simulink model "SecRwLtStBkReclnIsPosChk"  (R2024b)
settings: Solver=FixedStepDiscrete  StartTime=0.0  StopTime=10.0  FixedStep=0.01  RelTol=1e-3
undefined symbols (not defined in the file or in its folder): KeSMSuSecRwStBackPosDelta_Val, KeSMSuSecRwStBackPosTolr_Val, KeSMSuVehicleModelConfig_Val
libraries: StIsPosChkLib x13, simulink x7
(part 1 of 2)
settings Model: Creator=sn2xws  LastModifiedBy=sn55gm
settings Model: ModifiedHistory=|
  | 2023.8.1 V2.0.0 CR421790 增加模式21-26
  | 2024.3.14
  | V2.3.0
  | Bug 813950 童锁Lock，Mode1_Easy Entry Mode 不应调用失败
  | 2024.5.7 557 eze模式变更
  | 2024.7.8 V3.0.1 557模式流程V1.9
  | 2024.8.20 V3.0.2 Md32isposZone不看二排靠背
  | 2024.9.4 V3.0.3 增加Md56大四座模式（替代MD25）注释掉不用的模式
  | 2024.9.18 V3.0.4 Md27误注释恢复
  | 2024.12.17 V3.0.5 Md57 Md58 报失败问题修复
  | 2025.5.20 V3.12.0 童锁 Md56应报成功
  | 25.7.1 V3.13.0 新增Md61 Md62
settings SolverCC: AlgebraicLoopSolver=TrustRegion
settings DataIOCC: SaveFormat=StructureWithTime  ReturnWorkspaceOutputs=off
settings OptimizationCC: DefaultParameterBehavior=Inlined  EnhancedBackFolding=on  PassReuseOutputArgsAs=Individual arguments  ZeroExternalMemoryAtStartup=off  ZeroInternalMemoryAtStartup=off  OptimizeBlockOrder=speed  DifferentSizesBufferReuse=on  OptimizationCustomize=off  EfficientTunableParamExpr=on
settings DebuggingCC: ParameterTunabilityLossMsg=error  UnconnectedInputMsg=warning  UnconnectedOutputMsg=warning  UnconnectedLineMsg=warning  ArithmeticOperatorsInVariantConditions=warning
settings ModelReferenceCC: EnableRefExpFcnMdlSchedulingChecks=on  ModelReferenceNumInstancesAllowed=Single
settings SFSimCC: MATLABDynamicMemAlloc=off  CustomCodeUndefinedFunction=UseInterfaceOnly
settings RTWCC: Description=AUTOSAR  SystemTargetFile=autosar.tlc  GenCodeOnly=on  TemplateMakefile=ert_default_tmf  GenerateReport=on  IncludeHyperlinkInReport=on  LaunchReport=on  DataTypeReplacement=CDataTypesFixedWidth  GenerateTraceInfo=on  GenerateTraceReport=on  GenerateTraceReportSl=on  GenerateTraceReportSf=on  GenerateTraceReportEml=on  GenerateCodeMetricsReport=on  GPUComputeCapability=3.5
settings CodeAppCC: ForceParamTrailComments=on  IgnoreCustomStorageClasses=off  OperatorAnnotations=on  SimulinkDataObjDesc=on  SFDataObjDesc=on  InsertBlockDesc=on
settings STFCustomTargetCC: TargetLangStandard=C99 (ISO)  MultiwordLength=256  ParMdlRefBuildCompliant=on  CompOptLevelCompliant=on  IncludeMdlTerminateFcn=off  CombineOutputUpdateFcns=on  SuppressErrorStatus=on  ERTCustomFileBanners=on  SupportNonFinite=off  SupportComplex=off  SupportContinuousTime=off  SupportNonInlinedSFcns=off  RemoveResetFunc=on  MATLABClassNameForMDSCustomization=Simulink.SoftwareTarget.ERTCustomization  AutosarCompliant=on  UseToolchainInfoCompliant=on  LookupTableObjectStructAxisOrder=2,1,3,4,...  LUTObjectStructOrderEvenSpacing=Size,Table,Breakpoints  SystemTargetFile=autosar.tlc
settings ERTTargetCC: TargetLangStandard=C99 (ISO)  ConcurrentExecutionCompliant=off  IncludeMdlTerminateFcn=off  SuppressErrorStatus=on  SupportNonFinite=off  SupportComplex=off  ModelStepFunctionPrototypeControlCompliant=off  CPPClassGenCompliant=off  AutosarCompliant=on  LookupTableObjectStructAxisOrder=2,1,3,4,...  LUTObjectStructOrderEvenSpacing=Size,Table,Breakpoints  ERTCustomFileTemplate=example_file_process.tlc  ERTFilePackagingFormat=Compact  BooleanTrueId=TRUE  BooleanFalseId=FALSE  DynamicArrayContainerType=coder::array

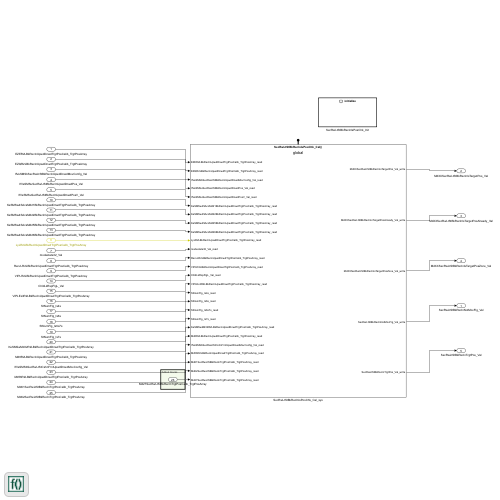
[thumbnail: Simulink's stored preview of the top-level diagram]
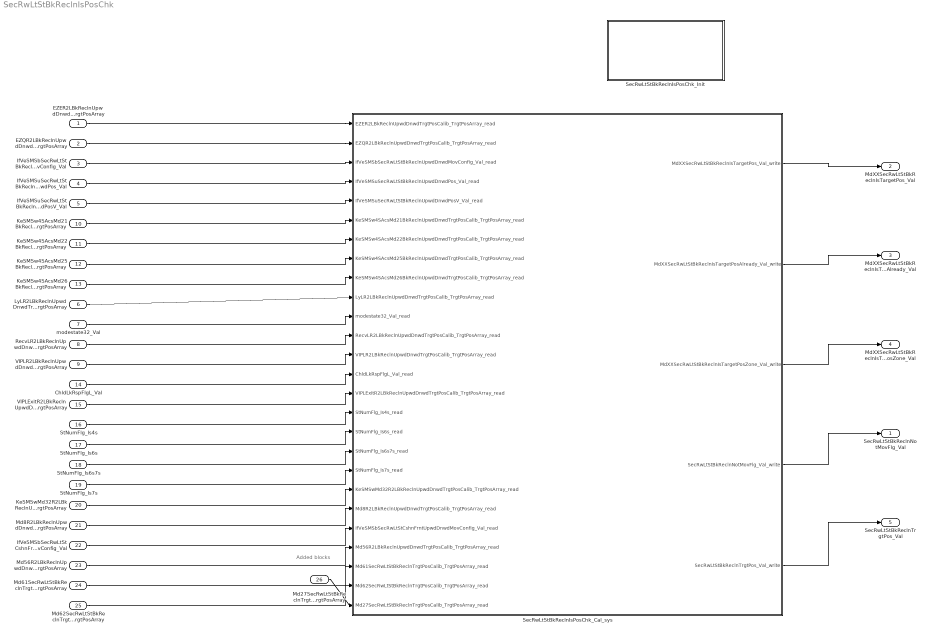
== system SecRwLtStBkReclnIsPosChk ==
  note: Added blocks
  EZER2LBkReclnUpwdDnwdTrgtPosCalib_TrgtPosArray : Inport  Description=|  OutDataTypeStr=uint16  PortDimensions=3
      | 0:Pos
      | 1:Max
      | 2:Min
  EZQR2LBkReclnUpwdDnwdTrgtPosCalib_TrgtPosArray : Inport  Description=|  Port=2  OutDataTypeStr=uint16  PortDimensions=3
      | 0:Pos
      | 1:Max
      | 2:Min
  IfVeSMSbSecRwLtStBkReclnUpwdDnwdMovConfig_Val : Inport  Port=3  OutDataTypeStr=boolean  PortDimensions=1
  IfVeSMSuSecRwLtStBkReclnUpwdDnwdPos_Val : Inport  Port=4  OutDataTypeStr=uint16  PortDimensions=1
  IfVeSMSuSecRwLtStBkReclnUpwdDnwdPosV_Val : Inport  Port=5  OutDataTypeStr=boolean  PortDimensions=1
  LyLR2LBkReclnUpwdDnwdTrgtPosCalib_TrgtPosArray : Inport  Description=|  Port=6  OutDataTypeStr=uint16  PortDimensions=3
      | 0:Pos
      | 1:Max
      | 2:Min
  modestate32_Val : Inport  Port=7  OutDataTypeStr=uint32  PortDimensions=1
  RecvLR2LBkReclnUpwdDnwdTrgtPosCalib_TrgtPosArray : Inport  Description=|  Port=8  OutDataTypeStr=uint16  PortDimensions=3
      | 0:Pos
      | 1:Max
      | 2:Min
  VIPLR2LBkReclnUpwdDnwdTrgtPosCalib_TrgtPosArray : Inport  Description=|  Port=9  OutDataTypeStr=uint16  PortDimensions=3
      | 0:Pos
      | 1:Max
      | 2:Min
  KeSMSw4SAcsMd21BkReclnUpwdDnwdTrgtPosCalib_TrgtPosArray : Inport  Description=|  Port=10  OutDataTypeStr=uint16  PortDimensions=3
      | 0:Pos
      | 1:Max
      | 2:Min
  KeSMSw4SAcsMd22BkReclnUpwdDnwdTrgtPosCalib_TrgtPosArray : Inport  Description=|  Port=11  OutDataTypeStr=uint16  PortDimensions=3
      | 0:Pos
      | 1:Max
      | 2:Min
  KeSMSw4SAcsMd25BkReclnUpwdDnwdTrgtPosCalib_TrgtPosArray : Inport  Description=|  Port=12  OutDataTypeStr=uint16  PortDimensions=3
      | 0:Pos
      | 1:Max
      | 2:Min
  KeSMSw4SAcsMd26BkReclnUpwdDnwdTrgtPosCalib_TrgtPosArray : Inport  Description=|  Port=13  OutDataTypeStr=uint16  PortDimensions=3
      | 0:Pos
      | 1:Max
      | 2:Min
  ChldLkRspFlgL_Val : Inport  Port=14  OutDataTypeStr=boolean  PortDimensions=1
  VIPLExitR2LBkReclnUpwdDnwdTrgtPosCalib_TrgtPosArray : Inport  Description=|  Port=15  OutDataTypeStr=uint16  PortDimensions=3
      | 0:Pos
      | 1:Max
      | 2:Min
  StNumFlg_Is4s : Inport  Port=16  OutDataTypeStr=boolean  PortDimensions=1
  StNumFlg_Is6s : Inport  Port=17  OutDataTypeStr=boolean  PortDimensions=1
  StNumFlg_Is6s7s : Inport  Port=18  OutDataTypeStr=boolean  PortDimensions=1
  StNumFlg_Is7s : Inport  Port=19  OutDataTypeStr=boolean  PortDimensions=1
  KeSMSwMd32R2LBkReclnUpwdDnwdTrgtPosCalib_TrgtPosArray : Inport  Description=|  Port=20  OutDataTypeStr=uint16  PortDimensions=3
      | 0:Pos
      | 1:Max
      | 2:Min
  Md8R2LBkReclnUpwdDnwdTrgtPosCalib_TrgtPosArray : Inport  Description=|  Port=21  OutDataTypeStr=uint16  PortDimensions=3
      | 0:Pos
      | 1:Max
      | 2:Min
  IfVeSMSbSecRwLtStCshnFrntUpwdDnwdMovConfig_Val : Inport  Port=22  OutDataTypeStr=boolean  PortDimensions=1
  Md56R2LBkReclnUpwdDnwdTrgtPosCalib_TrgtPosArray : Inport  Description=|  Port=23  OutDataTypeStr=uint16  PortDimensions=3
      | 0:Pos
      | 1:Max
      | 2:Min
  Md61SecRwLtStBkReclnTrgtPosCalib_TrgtPosArray : Inport  Description=|  Port=24  OutDataTypeStr=uint16  PortDimensions=3
      | 0:Pos
      | 1:Max
      | 2:Min
  Md62SecRwLtStBkReclnTrgtPosCalib_TrgtPosArray : Inport  Description=|  Port=25  OutDataTypeStr=uint16  PortDimensions=3
      | 0:Pos
      | 1:Max
      | 2:Min
  Md27SecRwLtStBkReclnTrgtPosCalib_TrgtPosArray : Inport  Description=|  Port=26  OutDataTypeStr=uint16  PortDimensions=3
      | 0:Pos
      | 1:Max
      | 2:Min
  SecRwLtStBkReclnIsPosChk_Cal_sys : Subsystem
  SecRwLtStBkReclnIsPosChk_Init : Subsystem
  SecRwLtStBkReclnNotMovFlg_Val : Outport  OutDataTypeStr=boolean  PortDimensions=1  VectorParamsAs1DForOutWhenUnconnected=off
  MdXXSecRwLtStBkReclnIsTargetPos_Val : Outport  Port=2  OutDataTypeStr=uint32  PortDimensions=1  VectorParamsAs1DForOutWhenUnconnected=off
  MdXXSecRwLtStBkReclnIsTargetPosAlready_Val : Outport  Port=3  OutDataTypeStr=uint32  PortDimensions=1  VectorParamsAs1DForOutWhenUnconnected=off
  MdXXSecRwLtStBkReclnIsTargetPosZone_Val : Outport  Port=4  OutDataTypeStr=uint32  PortDimensions=1  VectorParamsAs1DForOutWhenUnconnected=off
  SecRwLtStBkReclnTrgtPos_Val : Outport  Port=5  OutDataTypeStr=uint16  PortDimensions=1  VectorParamsAs1DForOutWhenUnconnected=off
  wires:
  EZER2LBkReclnUpwdDnwdTrgtPosCalib_TrgtPosArray/1 -> SecRwLtStBkReclnIsPosChk_Cal_sys/1(EZER2LBkReclnUpwdDnwdTrgtPosCalib_TrgtPosArray_read)
  EZQR2LBkReclnUpwdDnwdTrgtPosCalib_TrgtPosArray/1 -> SecRwLtStBkReclnIsPosChk_Cal_sys/2(EZQR2LBkReclnUpwdDnwdTrgtPosCalib_TrgtPosArray_read)
  IfVeSMSbSecRwLtStBkReclnUpwdDnwdMovConfig_Val/1 -> SecRwLtStBkReclnIsPosChk_Cal_sys/3(IfVeSMSbSecRwLtStBkReclnUpwdDnwdMovConfig_Val_read)
  IfVeSMSuSecRwLtStBkReclnUpwdDnwdPos_Val/1 -> SecRwLtStBkReclnIsPosChk_Cal_sys/4(IfVeSMSuSecRwLtStBkReclnUpwdDnwdPos_Val_read)
  IfVeSMSuSecRwLtStBkReclnUpwdDnwdPosV_Val/1 -> SecRwLtStBkReclnIsPosChk_Cal_sys/5(IfVeSMSuSecRwLtStBkReclnUpwdDnwdPosV_Val_read)
  LyLR2LBkReclnUpwdDnwdTrgtPosCalib_TrgtPosArray/1 -> SecRwLtStBkReclnIsPosChk_Cal_sys/10(LyLR2LBkReclnUpwdDnwdTrgtPosCalib_TrgtPosArray_read)
  modestate32_Val/1 -> SecRwLtStBkReclnIsPosChk_Cal_sys/11(modestate32_Val_read)
  RecvLR2LBkReclnUpwdDnwdTrgtPosCalib_TrgtPosArray/1 -> SecRwLtStBkReclnIsPosChk_Cal_sys/12(RecvLR2LBkReclnUpwdDnwdTrgtPosCalib_TrgtPosArray_read)
  VIPLR2LBkReclnUpwdDnwdTrgtPosCalib_TrgtPosArray/1 -> SecRwLtStBkReclnIsPosChk_Cal_sys/13(VIPLR2LBkReclnUpwdDnwdTrgtPosCalib_TrgtPosArray_read)
  SecRwLtStBkReclnIsPosChk_Cal_sys/1(MdXXSecRwLtStBkReclnIsTargetPos_Val_write) -> MdXXSecRwLtStBkReclnIsTargetPos_Val/1
  SecRwLtStBkReclnIsPosChk_Cal_sys/2(MdXXSecRwLtStBkReclnIsTargetPosAlready_Val_write) -> MdXXSecRwLtStBkReclnIsTargetPosAlready_Val/1
  SecRwLtStBkReclnIsPosChk_Cal_sys/3(MdXXSecRwLtStBkReclnIsTargetPosZone_Val_write) -> MdXXSecRwLtStBkReclnIsTargetPosZone_Val/1
  SecRwLtStBkReclnIsPosChk_Cal_sys/4(SecRwLtStBkReclnNotMovFlg_Val_write) -> SecRwLtStBkReclnNotMovFlg_Val/1
  SecRwLtStBkReclnIsPosChk_Cal_sys/5(SecRwLtStBkReclnTrgtPos_Val_write) -> SecRwLtStBkReclnTrgtPos_Val/1
  KeSMSw4SAcsMd21BkReclnUpwdDnwdTrgtPosCalib_TrgtPosArray/1 -> SecRwLtStBkReclnIsPosChk_Cal_sys/6(KeSMSw4SAcsMd21BkReclnUpwdDnwdTrgtPosCalib_TrgtPosArray_read)
  KeSMSw4SAcsMd22BkReclnUpwdDnwdTrgtPosCalib_TrgtPosArray/1 -> SecRwLtStBkReclnIsPosChk_Cal_sys/7(KeSMSw4SAcsMd22BkReclnUpwdDnwdTrgtPosCalib_TrgtPosArray_read)
  KeSMSw4SAcsMd25BkReclnUpwdDnwdTrgtPosCalib_TrgtPosArray/1 -> SecRwLtStBkReclnIsPosChk_Cal_sys/8(KeSMSw4SAcsMd25BkReclnUpwdDnwdTrgtPosCalib_TrgtPosArray_read)
  KeSMSw4SAcsMd26BkReclnUpwdDnwdTrgtPosCalib_TrgtPosArray/1 -> SecRwLtStBkReclnIsPosChk_Cal_sys/9(KeSMSw4SAcsMd26BkReclnUpwdDnwdTrgtPosCalib_TrgtPosArray_read)
  ChldLkRspFlgL_Val/1 -> SecRwLtStBkReclnIsPosChk_Cal_sys/14(ChldLkRspFlgL_Val_read)
  VIPLExitR2LBkReclnUpwdDnwdTrgtPosCalib_TrgtPosArray/1 -> SecRwLtStBkReclnIsPosChk_Cal_sys/15(VIPLExitR2LBkReclnUpwdDnwdTrgtPosCalib_TrgtPosArray_read)
  StNumFlg_Is4s/1 -> SecRwLtStBkReclnIsPosChk_Cal_sys/16(StNumFlg_Is4s_read)
  StNumFlg_Is6s/1 -> SecRwLtStBkReclnIsPosChk_Cal_sys/17(StNumFlg_Is6s_read)
  StNumFlg_Is6s7s/1 -> SecRwLtStBkReclnIsPosChk_Cal_sys/18(StNumFlg_Is6s7s_read)
  StNumFlg_Is7s/1 -> SecRwLtStBkReclnIsPosChk_Cal_sys/19(StNumFlg_Is7s_read)
  KeSMSwMd32R2LBkReclnUpwdDnwdTrgtPosCalib_TrgtPosArray/1 -> SecRwLtStBkReclnIsPosChk_Cal_sys/20(KeSMSwMd32R2LBkReclnUpwdDnwdTrgtPosCalib_TrgtPosArray_read)
  Md8R2LBkReclnUpwdDnwdTrgtPosCalib_TrgtPosArray/1 -> SecRwLtStBkReclnIsPosChk_Cal_sys/21(Md8R2LBkReclnUpwdDnwdTrgtPosCalib_TrgtPosArray_read)
  IfVeSMSbSecRwLtStCshnFrntUpwdDnwdMovConfig_Val/1 -> SecRwLtStBkReclnIsPosChk_Cal_sys/22(IfVeSMSbSecRwLtStCshnFrntUpwdDnwdMovConfig_Val_read)
  Md56R2LBkReclnUpwdDnwdTrgtPosCalib_TrgtPosArray/1 -> SecRwLtStBkReclnIsPosChk_Cal_sys/23(Md56R2LBkReclnUpwdDnwdTrgtPosCalib_TrgtPosArray_read)
  Md61SecRwLtStBkReclnTrgtPosCalib_TrgtPosArray/1 -> SecRwLtStBkReclnIsPosChk_Cal_sys/24(Md61SecRwLtStBkReclnTrgtPosCalib_TrgtPosArray_read)
  Md62SecRwLtStBkReclnTrgtPosCalib_TrgtPosArray/1 -> SecRwLtStBkReclnIsPosChk_Cal_sys/25(Md62SecRwLtStBkReclnTrgtPosCalib_TrgtPosArray_read)
  Md27SecRwLtStBkReclnTrgtPosCalib_TrgtPosArray/1 -> SecRwLtStBkReclnIsPosChk_Cal_sys/26(Md27SecRwLtStBkReclnTrgtPosCalib_TrgtPosArray_read)

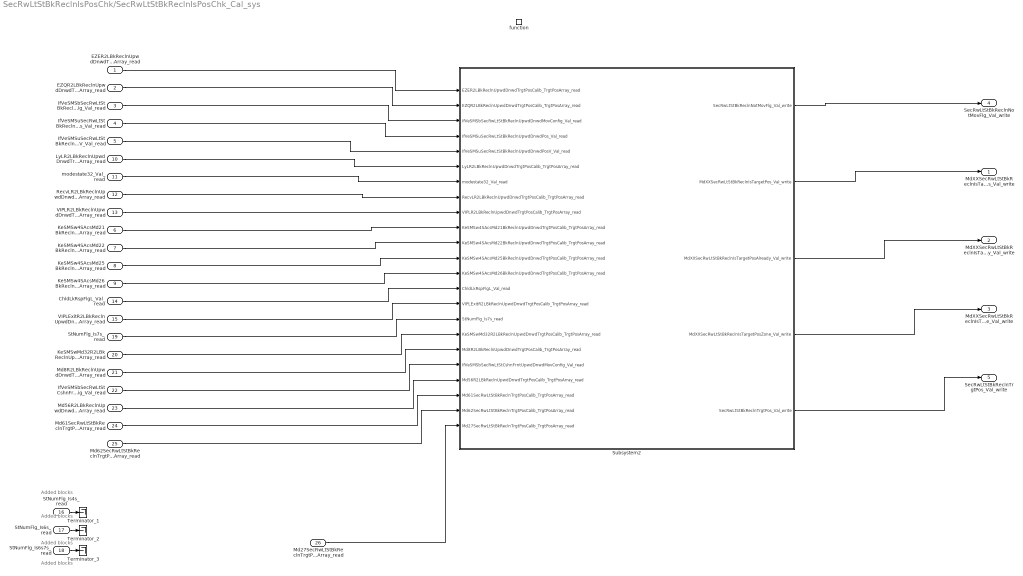
== system SecRwLtStBkReclnIsPosChk/SecRwLtStBkReclnIsPosChk_Cal_sys ==
  note: Added blocks
  note: Added blocks
  note: Added blocks
  note: Added blocks
  EZER2LBkReclnUpwdDnwdTrgtPosCalib_TrgtPosArray_read : Inport
  EZQR2LBkReclnUpwdDnwdTrgtPosCalib_TrgtPosArray_read : Inport  Port=2
  IfVeSMSbSecRwLtStBkReclnUpwdDnwdMovConfig_Val_read : Inport  Port=3
  IfVeSMSuSecRwLtStBkReclnUpwdDnwdPos_Val_read : Inport  Port=4
  IfVeSMSuSecRwLtStBkReclnUpwdDnwdPosV_Val_read : Inport  Port=5
  KeSMSw4SAcsMd21BkReclnUpwdDnwdTrgtPosCalib_TrgtPosArray_read : Inport  Port=6
  KeSMSw4SAcsMd22BkReclnUpwdDnwdTrgtPosCalib_TrgtPosArray_read : Inport  Port=7
  KeSMSw4SAcsMd25BkReclnUpwdDnwdTrgtPosCalib_TrgtPosArray_read : Inport  Port=8
  KeSMSw4SAcsMd26BkReclnUpwdDnwdTrgtPosCalib_TrgtPosArray_read : Inport  Port=9
  LyLR2LBkReclnUpwdDnwdTrgtPosCalib_TrgtPosArray_read : Inport  Port=10
  modestate32_Val_read : Inport  Port=11
  RecvLR2LBkReclnUpwdDnwdTrgtPosCalib_TrgtPosArray_read : Inport  Port=12
  VIPLR2LBkReclnUpwdDnwdTrgtPosCalib_TrgtPosArray_read : Inport  Port=13
  ChldLkRspFlgL_Val_read : Inport  Port=14
  VIPLExitR2LBkReclnUpwdDnwdTrgtPosCalib_TrgtPosArray_read : Inport  Port=15
  StNumFlg_Is4s_read : Inport  Port=16
  StNumFlg_Is6s_read : Inport  Port=17
  StNumFlg_Is6s7s_read : Inport  Port=18
  StNumFlg_Is7s_read : Inport  Port=19
  KeSMSwMd32R2LBkReclnUpwdDnwdTrgtPosCalib_TrgtPosArray_read : Inport  Port=20
  Md8R2LBkReclnUpwdDnwdTrgtPosCalib_TrgtPosArray_read : Inport  Port=21
  IfVeSMSbSecRwLtStCshnFrntUpwdDnwdMovConfig_Val_read : Inport  Port=22
  Md56R2LBkReclnUpwdDnwdTrgtPosCalib_TrgtPosArray_read : Inport  Port=23
  Md61SecRwLtStBkReclnTrgtPosCalib_TrgtPosArray_read : Inport  Port=24
  Md62SecRwLtStBkReclnTrgtPosCalib_TrgtPosArray_read : Inport  Port=25
  Md27SecRwLtStBkReclnTrgtPosCalib_TrgtPosArray_read : Inport  Port=26
  function : TriggerPort  TriggerType=function-call  IsSimulinkFunction=on  FunctionName=SecRwLtStBkReclnIsPosChk_Cal  VariantControl=(inherit)
  Subsystem2 : Subsystem
  Terminator_1 : Terminator
  Terminator_2 : Terminator
  Terminator_3 : Terminator
  MdXXSecRwLtStBkReclnIsTargetPos_Val_write : Outport  VectorParamsAs1DForOutWhenUnconnected=off
      settings: EnsureOutportIsVirtual=on
  MdXXSecRwLtStBkReclnIsTargetPosAlready_Val_write : Outport  Port=2  VectorParamsAs1DForOutWhenUnconnected=off
      settings: EnsureOutportIsVirtual=on
  MdXXSecRwLtStBkReclnIsTargetPosZone_Val_write : Outport  Port=3  VectorParamsAs1DForOutWhenUnconnected=off
      settings: EnsureOutportIsVirtual=on
  SecRwLtStBkReclnNotMovFlg_Val_write : Outport  Port=4  VectorParamsAs1DForOutWhenUnconnected=off
      settings: EnsureOutportIsVirtual=on
  SecRwLtStBkReclnTrgtPos_Val_write : Outport  Port=5  VectorParamsAs1DForOutWhenUnconnected=off
      settings: EnsureOutportIsVirtual=on
  wires:
  Subsystem2/1(SecRwLtStBkReclnNotMovFlg_Val_write) -> SecRwLtStBkReclnNotMovFlg_Val_write/1
  Subsystem2/2(MdXXSecRwLtStBkReclnIsTargetPos_Val_write) -> MdXXSecRwLtStBkReclnIsTargetPos_Val_write/1
  Subsystem2/3(MdXXSecRwLtStBkReclnIsTargetPosAlready_Val_write) -> MdXXSecRwLtStBkReclnIsTargetPosAlready_Val_write/1
  Subsystem2/4(MdXXSecRwLtStBkReclnIsTargetPosZone_Val_write) -> MdXXSecRwLtStBkReclnIsTargetPosZone_Val_write/1
  Subsystem2/5(SecRwLtStBkReclnTrgtPos_Val_write) -> SecRwLtStBkReclnTrgtPos_Val_write/1
  EZER2LBkReclnUpwdDnwdTrgtPosCalib_TrgtPosArray_read/1 -> Subsystem2/1(EZER2LBkReclnUpwdDnwdTrgtPosCalib_TrgtPosArray_read)
  EZQR2LBkReclnUpwdDnwdTrgtPosCalib_TrgtPosArray_read/1 -> Subsystem2/2(EZQR2LBkReclnUpwdDnwdTrgtPosCalib_TrgtPosArray_read)
  IfVeSMSbSecRwLtStBkReclnUpwdDnwdMovConfig_Val_read/1 -> Subsystem2/3(IfVeSMSbSecRwLtStBkReclnUpwdDnwdMovConfig_Val_read)
  IfVeSMSuSecRwLtStBkReclnUpwdDnwdPos_Val_read/1 -> Subsystem2/4(IfVeSMSuSecRwLtStBkReclnUpwdDnwdPos_Val_read)
  IfVeSMSuSecRwLtStBkReclnUpwdDnwdPosV_Val_read/1 -> Subsystem2/5(IfVeSMSuSecRwLtStBkReclnUpwdDnwdPosV_Val_read)
  LyLR2LBkReclnUpwdDnwdTrgtPosCalib_TrgtPosArray_read/1 -> Subsystem2/6(LyLR2LBkReclnUpwdDnwdTrgtPosCalib_TrgtPosArray_read)
  modestate32_Val_read/1 -> Subsystem2/7(modestate32_Val_read)
  RecvLR2LBkReclnUpwdDnwdTrgtPosCalib_TrgtPosArray_read/1 -> Subsystem2/8(RecvLR2LBkReclnUpwdDnwdTrgtPosCalib_TrgtPosArray_read)
  VIPLR2LBkReclnUpwdDnwdTrgtPosCalib_TrgtPosArray_read/1 -> Subsystem2/9(VIPLR2LBkReclnUpwdDnwdTrgtPosCalib_TrgtPosArray_read)
  KeSMSw4SAcsMd21BkReclnUpwdDnwdTrgtPosCalib_TrgtPosArray_read/1 -> Subsystem2/10(KeSMSw4SAcsMd21BkReclnUpwdDnwdTrgtPosCalib_TrgtPosArray_read)
  KeSMSw4SAcsMd22BkReclnUpwdDnwdTrgtPosCalib_TrgtPosArray_read/1 -> Subsystem2/11(KeSMSw4SAcsMd22BkReclnUpwdDnwdTrgtPosCalib_TrgtPosArray_read)
  KeSMSw4SAcsMd25BkReclnUpwdDnwdTrgtPosCalib_TrgtPosArray_read/1 -> Subsystem2/12(KeSMSw4SAcsMd25BkReclnUpwdDnwdTrgtPosCalib_TrgtPosArray_read)
  KeSMSw4SAcsMd26BkReclnUpwdDnwdTrgtPosCalib_TrgtPosArray_read/1 -> Subsystem2/13(KeSMSw4SAcsMd26BkReclnUpwdDnwdTrgtPosCalib_TrgtPosArray_read)
  ChldLkRspFlgL_Val_read/1 -> Subsystem2/14(ChldLkRspFlgL_Val_read)
  VIPLExitR2LBkReclnUpwdDnwdTrgtPosCalib_TrgtPosArray_read/1 -> Subsystem2/15(VIPLExitR2LBkReclnUpwdDnwdTrgtPosCalib_TrgtPosArray_read)
  StNumFlg_Is4s_read/1 -> Terminator_1/1
  StNumFlg_Is6s_read/1 -> Terminator_2/1
  StNumFlg_Is6s7s_read/1 -> Terminator_3/1
  StNumFlg_Is7s_read/1 -> Subsystem2/16(StNumFlg_Is7s_read)
  KeSMSwMd32R2LBkReclnUpwdDnwdTrgtPosCalib_TrgtPosArray_read/1 -> Subsystem2/17(KeSMSwMd32R2LBkReclnUpwdDnwdTrgtPosCalib_TrgtPosArray_read)
  Md8R2LBkReclnUpwdDnwdTrgtPosCalib_TrgtPosArray_read/1 -> Subsystem2/18(Md8R2LBkReclnUpwdDnwdTrgtPosCalib_TrgtPosArray_read)
  IfVeSMSbSecRwLtStCshnFrntUpwdDnwdMovConfig_Val_read/1 -> Subsystem2/19(IfVeSMSbSecRwLtStCshnFrntUpwdDnwdMovConfig_Val_read)
  Md56R2LBkReclnUpwdDnwdTrgtPosCalib_TrgtPosArray_read/1 -> Subsystem2/20(Md56R2LBkReclnUpwdDnwdTrgtPosCalib_TrgtPosArray_read)
  Md61SecRwLtStBkReclnTrgtPosCalib_TrgtPosArray_read/1 -> Subsystem2/21(Md61SecRwLtStBkReclnTrgtPosCalib_TrgtPosArray_read)
  Md62SecRwLtStBkReclnTrgtPosCalib_TrgtPosArray_read/1 -> Subsystem2/22(Md62SecRwLtStBkReclnTrgtPosCalib_TrgtPosArray_read)
  Md27SecRwLtStBkReclnTrgtPosCalib_TrgtPosArray_read/1 -> Subsystem2/23(Md27SecRwLtStBkReclnTrgtPosCalib_TrgtPosArray_read)

== system SecRwLtStBkReclnIsPosChk/SecRwLtStBkReclnIsPosChk_Init ==
  note: Added blocks
  Event Listener : EventListener  EventName=reset
  PA_KeSMSuSecRwStBackPosDelta_Val : Constant  Value=KeSMSuSecRwStBackPosDelta_Val
  PA_KeSMSuSecRwStBackPosTolr_Val : Constant  Value=KeSMSuSecRwStBackPosTolr_Val
  PA_KeSMSuVehicleModelConfig_Val : Constant  Value=KeSMSuVehicleModelConfig_Val
  Terminator_1 : Terminator
  Terminator_2 : Terminator
  Terminator_4 : Terminator
  wires:
  PA_KeSMSuSecRwStBackPosDelta_Val/1 -> Terminator_1/1
  PA_KeSMSuSecRwStBackPosTolr_Val/1 -> Terminator_2/1
  PA_KeSMSuVehicleModelConfig_Val/1 -> Terminator_4/1

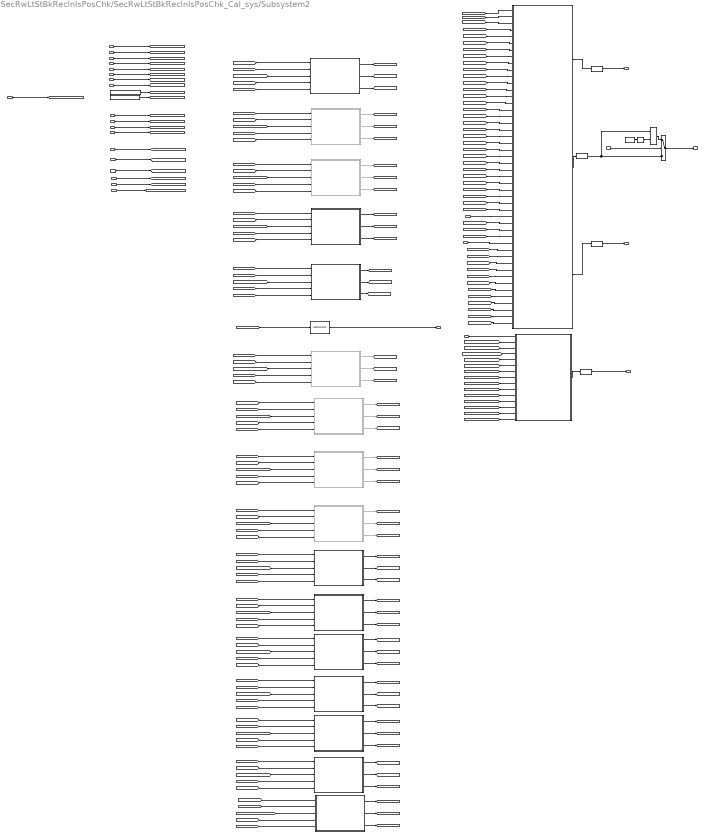
== system SecRwLtStBkReclnIsPosChk/SecRwLtStBkReclnIsPosChk_Cal_sys/Subsystem2 ==
  note: 2023.8.1 V2.0.0 CR421790 增加模式21-26
  EZER2LBkReclnUpwdDnwdTrgtPosCalib_TrgtPosArray_read : Inport
  EZQR2LBkReclnUpwdDnwdTrgtPosCalib_TrgtPosArray_read : Inport  Port=2
  IfVeSMSbSecRwLtStBkReclnUpwdDnwdMovConfig_Val_read : Inport  Port=3
  IfVeSMSuSecRwLtStBkReclnUpwdDnwdPos_Val_read : Inport  Port=4
  IfVeSMSuSecRwLtStBkReclnUpwdDnwdPosV_Val_read : Inport  Port=5
  LyLR2LBkReclnUpwdDnwdTrgtPosCalib_TrgtPosArray_read : Inport  Port=6
  modestate32_Val_read : Inport  Port=7
  RecvLR2LBkReclnUpwdDnwdTrgtPosCalib_TrgtPosArray_read : Inport  Port=8
  VIPLR2LBkReclnUpwdDnwdTrgtPosCalib_TrgtPosArray_read : Inport  Port=9
  KeSMSw4SAcsMd21BkReclnUpwdDnwdTrgtPosCalib_TrgtPosArray_read : Inport  Port=10
  KeSMSw4SAcsMd22BkReclnUpwdDnwdTrgtPosCalib_TrgtPosArray_read : Inport  Port=11
  KeSMSw4SAcsMd25BkReclnUpwdDnwdTrgtPosCalib_TrgtPosArray_read : Inport  Port=12
  KeSMSw4SAcsMd26BkReclnUpwdDnwdTrgtPosCalib_TrgtPosArray_read : Inport  Port=13
  ChldLkRspFlgL_Val_read : Inport  Port=14
  VIPLExitR2LBkReclnUpwdDnwdTrgtPosCalib_TrgtPosArray_read : Inport  Port=15
  StNumFlg_Is7s_read : Inport  Port=16
  KeSMSwMd32R2LBkReclnUpwdDnwdTrgtPosCalib_TrgtPosArray_read : Inport  Port=17
  Md8R2LBkReclnUpwdDnwdTrgtPosCalib_TrgtPosArray_read : Inport  Port=18
  IfVeSMSbSecRwLtStCshnFrntUpwdDnwdMovConfig_Val_read : Inport  Port=19
  Md56R2LBkReclnUpwdDnwdTrgtPosCalib_TrgtPosArray_read : Inport  Port=20
  Md61SecRwLtStBkReclnTrgtPosCalib_TrgtPosArray_read : Inport  Port=21
  Md62SecRwLtStBkReclnTrgtPosCalib_TrgtPosArray_read : Inport  Port=22
  Md27SecRwLtStBkReclnTrgtPosCalib_TrgtPosArray_read : Inport  Port=23
  Bitwise Operator : simulink/Logic and Bit Operations/Bitwise Operator  logicop=AND  UseBitMask=off  NumInputPorts=2  BitMask=bin2dec('11011001')  BitMaskRealWorld=Stored Integer
  Bitwise Operator1 : simulink/Logic and Bit Operations/Bitwise Operator  logicop=NOT  UseBitMask=off  BitMask=bin2dec('11011001')  BitMaskRealWorld=Stored Integer
  Constant : Constant  Value=512  OutDataTypeStr=uint32
  Data Type Conversion{,1..3} (4 alike) : DataTypeConversion  SaturateOnIntegerOverflow=off  RndMeth=Floor
  NotMovChk : StIsPosChkLib/NotMovChk  SystemSampleTime=-1  VariantActivationTime=update diagram  AllowFlexibleInterface=on  Latency=0  AutoFrameSizeCalculation=off
  PA_KeSMSuSecRwStBackPosDelta_Val : Constant  Value=KeSMSuSecRwStBackPosDelta_Val
  PA_KeSMSuSecRwStBackPosTolr_Val : Constant  Value=KeSMSuSecRwStBackPosTolr_Val
  Subsystem : Subsystem
  Subsystem1 : Subsystem
  Subsystem10 : Subsystem  Commented=on
  Subsystem11 : Subsystem
  Subsystem12 : Subsystem
  Subsystem13 : Subsystem
  Subsystem14 : Subsystem
  Subsystem15 : Subsystem
  Subsystem16 : Subsystem
  Subsystem17 : Subsystem
  Subsystem2 : Subsystem
  Subsystem3 : Subsystem  Commented=on
  Subsystem4 : Subsystem  Commented=on
  Subsystem5 : Subsystem
  Subsystem6 : Subsystem
  Subsystem7 : Subsystem  Commented=on
  Subsystem8 : Subsystem  Commented=on
  Subsystem9 : Subsystem  Commented=on
  Switch : Switch  Criteria=u2 > Threshold  SaturateOnIntegerOverflow=off  InputSameDT=off
  SecRwLtStBkReclnNotMovFlg_Val_write : Outport  VectorParamsAs1DForOutWhenUnconnected=off
      settings: EnsureOutportIsVirtual=on
  MdXXSecRwLtStBkReclnIsTargetPos_Val_write : Outport  Port=2  VectorParamsAs1DForOutWhenUnconnected=off
      settings: EnsureOutportIsVirtual=on
  MdXXSecRwLtStBkReclnIsTargetPosAlready_Val_write : Outport  Port=3  VectorParamsAs1DForOutWhenUnconnected=off
      settings: EnsureOutportIsVirtual=on
  MdXXSecRwLtStBkReclnIsTargetPosZone_Val_write : Outport  Port=4  VectorParamsAs1DForOutWhenUnconnected=off
      settings: EnsureOutportIsVirtual=on
  SecRwLtStBkReclnTrgtPos_Val_write : Outport  Port=5  VectorParamsAs1DForOutWhenUnconnected=off
      settings: EnsureOutportIsVirtual=on
  wires:
  [VIPLCalib] -> Subsystem6/3(CalibArray)
  [PosDelta] -> Subsystem3/4(Delta)
  Subsystem6/2(IsPosZone) -> [VIPLIsTargetPosZone]
  [LyLIsTargetPosZone] -> Subsystem1/17(LyLIsTargetPosZone)
  [EZEIsTargetPos] -> Subsystem1/5(EZEIsTargetPos)
  [LyLIsTargetPos] -> Subsystem1/7(LyLIsTargetPos)
  Subsystem4/3(IsPosAlready) -> [LyLIsTargetPosAlready]
  Subsystem4/2(IsPosZone) -> [LyLIsTargetPosZone]
  [RecvLCalib] -> Subsystem5/3(CalibArray)
  [Pos] -> Subsystem6/2(Pos)
  VIPLR2LBkReclnUpwdDnwdTrgtPosCalib_TrgtPosArray_read/1 -> [VIPLCalib]
  PA_KeSMSuSecRwStBackPosDelta_Val/1 -> [PosDelta]
  [EZEIsTargetPosAlready] -> Subsystem1/10(EZEIsTargetPosAlready)
  [Pos] -> NotMovChk/1
  Data Type Conversion/1 -> SecRwLtStBkReclnTrgtPos_Val_write/1
  Subsystem5/2(IsPosZone) -> [RecvLIsTargetPosZone]
  [PosV] -> Subsystem2/1(PosV)
  Subsystem1/2(IsTargetPosAlready) -> Data Type Conversion2/1
  [EZEIsTargetPosZone] -> Subsystem1/15(EZEIsTargetPosZone)
  [Pos] -> Subsystem3/2(Pos)
  [EZQIsTargetPosZone] -> Subsystem1/16(EZQIsTargetPosZone)
  IfVeSMSuSecRwLtStBkReclnUpwdDnwdPosV_Val_read/1 -> [PosV]
  Subsystem/1(TrgtPos) -> Data Type Conversion/1
  Subsystem3/1(IsPos) -> [EZQIsTargetPos]
  [VIPLCalib] -> Subsystem/6(VIPLCalib)
  [RecvLIsTargetPos] -> Subsystem1/8(RecvLIsTargetPos)
  [VIPLIsTargetPos] -> Subsystem1/9(VIPLIsTargetPos)
  IfVeSMSbSecRwLtStBkReclnUpwdDnwdMovConfig_Val_read/1 -> [MovConfig]
  [EZQCalib] -> Subsystem3/3(CalibArray)
  PA_KeSMSuSecRwStBackPosTolr_Val/1 -> [PosTolr]
  Subsystem5/3(IsPosAlready) -> [RecvLIsTargetPosAlready]
  [PosV] -> Subsystem3/1(PosV)
  [RecvLIsTargetPosZone] -> Subsystem1/18(RecvLIsTargetPosZone)
  IfVeSMSuSecRwLtStBkReclnUpwdDnwdPos_Val_read/1 -> [Pos]
  [PosDelta] -> Subsystem2/4(Delta)
  [Pos] -> Subsystem5/2(Pos)
  EZQR2LBkReclnUpwdDnwdTrgtPosCalib_TrgtPosArray_read/1 -> [EZQCalib]
  modestate32_Val_read/1 -> Subsystem/1(modestate32_Val_read)
  [PosTolr] -> Subsystem2/5(Tolr)
  [EZQIsTargetPosAlready] -> Subsystem1/11(EZQIsTargetPosAlready)
  [VIPLIsTargetPosAlready] -> Subsystem1/14(VIPLIsTargetPosAlready)
  [LyLIsTargetPosAlready] -> Subsystem1/12(LyLIsTargetPosAlready)
  [PosV] -> Subsystem6/1(PosV)
  [PosTolr] -> Subsystem5/5(Tolr)
  [VIPLIsTargetPosZone] -> Subsystem1/19(VIPLIsTargetPosZone)
  Subsystem1/3(IsTargetPosZone) -> Data Type Conversion3/1
  Data Type Conversion1/1 -> MdXXSecRwLtStBkReclnIsTargetPos_Val_write/1
  [LyLCalib] -> Subsystem4/3(CalibArray)
  Subsystem4/1(IsPos) -> [LyLIsTargetPos]
  Subsystem2/2(IsPosZone) -> [EZEIsTargetPosZone]
  [MovConfig] -> Subsystem1/4(MovConfig)
  [EZQIsTargetPos] -> Subsystem1/6(EZQIsTargetPos)
  [Pos] -> Subsystem4/2(Pos)
  Data Type Conversion3/1 -> MdXXSecRwLtStBkReclnIsTargetPosZone_Val_write/1
  Subsystem3/2(IsPosZone) -> [EZQIsTargetPosZone]
  EZER2LBkReclnUpwdDnwdTrgtPosCalib_TrgtPosArray_read/1 -> [EZECalib]
  [RecvLIsTargetPosAlready] -> Subsystem1/13(RecvLIsTargetPosAlready)
  RecvLR2LBkReclnUpwdDnwdTrgtPosCalib_TrgtPosArray_read/1 -> [RecvLCalib]
  Subsystem3/3(IsPosAlready) -> [EZQIsTargetPosAlready]
  [PosTolr] -> Subsystem4/5(Tolr)
  [PosV] -> Subsystem4/1(PosV)
  Subsystem5/1(IsPos) -> [RecvLIsTargetPos]
  [PosDelta] -> Subsystem4/4(Delta)
  [PosDelta] -> Subsystem6/4(Delta)
  Subsystem6/1(IsPos) -> [VIPLIsTargetPos]
  [PosTolr] -> Subsystem6/5(Tolr)
  [EZQCalib] -> Subsystem/3(EZQCalib)
  [PosTolr] -> Subsystem3/5(Tolr)
  [EZECalib] -> Subsystem/2(EZECalib)
  [RecvLCalib] -> Subsystem/5(RecvLCalib)
  [PosV] -> Subsystem5/1(PosV)
  LyLR2LBkReclnUpwdDnwdTrgtPosCalib_TrgtPosArray_read/1 -> [LyLCalib]
  [Md14Calib] -> Subsystem/4(LyLCalib)
  [PosDelta] -> Subsystem5/4(Delta)
  NotMovChk/1 -> SecRwLtStBkReclnNotMovFlg_Val_write/1
  Subsystem1/1(IsTargetPos) -> Data Type Conversion1/1
  [Pos] -> Subsystem2/2(Pos)
  Subsystem2/1(IsPos) -> [EZEIsTargetPos]
  [EZECalib] -> Subsystem2/3(CalibArray)
  Subsystem2/3(IsPosAlready) -> [EZEIsTargetPosAlready]
  KeSMSw4SAcsMd21BkReclnUpwdDnwdTrgtPosCalib_TrgtPosArray_read/1 -> [Md21Calib]
  KeSMSw4SAcsMd22BkReclnUpwdDnwdTrgtPosCalib_TrgtPosArray_read/1 -> [Md22Calib]
  KeSMSw4SAcsMd25BkReclnUpwdDnwdTrgtPosCalib_TrgtPosArray_read/1 -> [Md25Calib]
  KeSMSw4SAcsMd26BkReclnUpwdDnwdTrgtPosCalib_TrgtPosArray_read/1 -> [Md26Calib]
  [PosTolr] -> Subsystem7/5(Tolr)
  Subsystem7/3(IsPosAlready) -> [Md21IsTargetPosAlready]
  Subsystem7/1(IsPos) -> [Md21IsTargetPos]
  [PosDelta] -> Subsystem7/4(Delta)
  [PosV] -> Subsystem7/1(PosV)
  [Pos] -> Subsystem7/2(Pos)
  Subsystem7/2(IsPosZone) -> [Md21IsTargetPosZone]
  [Md21Calib] -> Subsystem7/3(CalibArray)
  [Md22Calib] -> Subsystem8/3(CalibArray)
  Subsystem8/2(IsPosZone) -> [Md22IsTargetPosZone]
  [Pos] -> Subsystem8/2(Pos)
  [PosV] -> Subsystem8/1(PosV)
  [PosDelta] -> Subsystem8/4(Delta)
  Subsystem8/1(IsPos) -> [Md22IsTargetPos]
  Subsystem8/3(IsPosAlready) -> [Md22IsTargetPosAlready]
  [PosTolr] -> Subsystem8/5(Tolr)
  [PosTolr] -> Subsystem9/5(Tolr)
  Subsystem9/3(IsPosAlready) -> [Md25IsTargetPosAlready]
  Subsystem9/1(IsPos) -> [Md25IsTargetPos]
  [PosDelta] -> Subsystem9/4(Delta)
  [PosV] -> Subsystem9/1(PosV)
  [Pos] -> Subsystem9/2(Pos)
  Subsystem9/2(IsPosZone) -> [Md25IsTargetPosZone]
  [Md25Calib] -> Subsystem9/3(CalibArray)
  [Md26Calib] -> Subsystem10/3(CalibArray)
  Subsystem10/2(IsPosZone) -> [Md26IsTargetPosZone]
  [Pos] -> Subsystem10/2(Pos)
  [PosV] -> Subsystem10/1(PosV)
  [PosDelta] -> Subsystem10/4(Delta)
  Subsystem10/1(IsPos) -> [Md26IsTargetPos]
  Subsystem10/3(IsPosAlready) -> [Md26IsTargetPosAlready]
  [PosTolr] -> Subsystem10/5(Tolr)
  [Md21Calib] -> Subsystem/7(Md21Calib)
  [Md22Calib] -> Subsystem/8(Md22Calib)
  [Md26Calib] -> Subsystem/10(Md26Calib)
  [Md21IsTargetPos] -> Subsystem1/20(Md21IsTargetPos)
  [Md22IsTargetPos] -> Subsystem1/21(Md22IsTargetPos)
  [Md56IsTargetPos] -> Subsystem1/22(Md25IsTargetPos)
  [Md26IsTargetPos] -> Subsystem1/23(Md26IsTargetPos)
  [Md21IsTargetPosAlready] -> Subsystem1/24(Md21IsTargetPosAlready)
  [Md22IsTargetPosAlready] -> Subsystem1/25(Md22IsTargetPosAlready)
  [Md56IsTargetPosAlready] -> Subsystem1/26(Md25IsTargetPosAlready)
  [Md26IsTargetPosAlready] -> Subsystem1/27(Md26IsTargetPosAlready)
  [Md21IsTargetPosZone] -> Subsystem1/28(Md21IsTargetPosZone)
  [Md22IsTargetPosZone] -> Subsystem1/29(Md22IsTargetPosZone)
  [Md56IsTargetPosZone] -> Subsystem1/30(Md25IsTargetPosZone)
  [Md26IsTargetPosZone] -> Subsystem1/31(Md26IsTargetPosZone)
  ChldLkRspFlgL_Val_read/1 -> Subsystem1/32(ChldLkRspFlgL_Val_read)
  [PosTolr] -> Subsystem11/5(Tolr)
  Subsystem11/3(IsPosAlready) -> [Md27IsTargetPosAlready]
  Subsystem11/1(IsPos) -> [Md27IsTargetPos]
  [PosDelta] -> Subsystem11/4(Delta)
  [PosV] -> Subsystem11/1(PosV)
  [Pos] -> Subsystem11/2(Pos)
  Subsystem11/2(IsPosZone) -> [Md27IsTargetPosZone]
  [Md27Calib] -> Subsystem11/3(CalibArray)
  [Md27Calib] -> Subsystem/11(Md27Calib)
  [Md27IsTargetPos] -> Subsystem1/33(Md27IsTargetPos)
  [Md27IsTargetPosAlready] -> Subsystem1/34(Md27IsTargetPosAlready)
  [Md27IsTargetPosZone] -> Subsystem1/35(Md27IsTargetPosZone)
  StNumFlg_Is7s_read/1 -> Subsystem1/36(StNumFlg_Is7s_read)
  KeSMSwMd32R2LBkReclnUpwdDnwdTrgtPosCalib_TrgtPosArray_read/1 -> [Md32Calib]
  [Md32Calib] -> Subsystem12/3(CalibArray)
  Subsystem12/2(IsPosZone) -> [Md32IsTargetPosZone]
  [Pos] -> Subsystem12/2(Pos)
  [PosV] -> Subsystem12/1(PosV)
  [PosDelta] -> Subsystem12/4(Delta)
  Subsystem12/1(IsPos) -> [Md32IsTargetPos]
  Subsystem12/3(IsPosAlready) -> [Md32IsTargetPosAlready]
  [PosTolr] -> Subsystem12/5(Tolr)
  [Md32Calib] -> Subsystem/12(Md32Calib)
  [Md32IsTargetPos] -> Subsystem1/37(Md32IsTargetPos)
  [Md32IsTargetPosAlready] -> Subsystem1/38(Md32IsTargetPosAlready)
  [Md32IsTargetPosZone] -> Subsystem1/39(Md32IsTargetPosZone)
  Md8R2LBkReclnUpwdDnwdTrgtPosCalib_TrgtPosArray_read/1 -> [Md8Calib]
  [PosTolr] -> Subsystem13/5(Tolr)
  Subsystem13/3(IsPosAlready) -> [Md8IsTargetPosAlready]
  Subsystem13/1(IsPos) -> [Md8IsTargetPos]
  [PosDelta] -> Subsystem13/4(Delta)
  [PosV] -> Subsystem13/1(PosV)
  [Pos] -> Subsystem13/2(Pos)
  Subsystem13/2(IsPosZone) -> [Md8IsTargetPosZone]
  [Md8Calib] -> Subsystem13/3(CalibArray)
  [Md8Calib] -> Subsystem/13(Md8Calib)
  [Md8IsTargetPos] -> Subsystem1/40(Md8IsTargetPos)
  [Md8IsTargetPosAlready] -> Subsystem1/41(Md8IsTargetPosAlready)
  [Md8IsTargetPosZone] -> Subsystem1/42(Md8IsTargetPosZone)
  Constant/1 -> Bitwise Operator1/1
  Bitwise Operator1/1 -> Bitwise Operator/2
  IfVeSMSbSecRwLtStCshnFrntUpwdDnwdMovConfig_Val_read/1 -> Switch/2
  Bitwise Operator/1 -> Switch/1
  Subsystem6/3(IsPosAlready) -> [VIPLIsTargetPosAlready]
  Data Type Conversion2/1 -> Switch/3, Bitwise Operator/1
  Switch/1 -> MdXXSecRwLtStBkReclnIsTargetPosAlready_Val_write/1
  Md56R2LBkReclnUpwdDnwdTrgtPosCalib_TrgtPosArray_read/1 -> [Md56Calib]
  [Md56Calib] -> Subsystem14/3(CalibArray)
  Subsystem14/2(IsPosZone) -> [Md56IsTargetPosZone]
  [Pos] -> Subsystem14/2(Pos)
  [PosV] -> Subsystem14/1(PosV)
  [PosDelta] -> Subsystem14/4(Delta)
  Subsystem14/1(IsPos) -> [Md56IsTargetPos]
  Subsystem14/3(IsPosAlready) -> [Md56IsTargetPosAlready]
  [PosTolr] -> Subsystem14/5(Tolr)
  [Md56Calib] -> Subsystem/9(Md25Calib)
  Md62SecRwLtStBkReclnTrgtPosCalib_TrgtPosArray_read/1 -> [Md62Calib]
  Md61SecRwLtStBkReclnTrgtPosCalib_TrgtPosArray_read/1 -> [Md61Calib]
  [PosTolr] -> Subsystem15/5(Tolr)
  Subsystem15/3(IsPosAlready) -> [Md61IsTargetPosAlready]
  Subsystem15/1(IsPos) -> [Md61IsTargetPos]
  [PosDelta] -> Subsystem15/4(Delta)
  [PosV] -> Subsystem15/1(PosV)
  [Pos] -> Subsystem15/2(Pos)
  Subsystem15/2(IsPosZone) -> [Md61IsTargetPosZone]
  [Md61Calib] -> Subsystem15/3(CalibArray)
  [Md62Calib] -> Subsystem16/3(CalibArray)
  Subsystem16/2(IsPosZone) -> [Md62IsTargetPosZone]
  [Pos] -> Subsystem16/2(Pos)
  [PosV] -> Subsystem16/1(PosV)
  [PosDelta] -> Subsystem16/4(Delta)
  Subsystem16/1(IsPos) -> [Md62IsTargetPos]
  Subsystem16/3(IsPosAlready) -> [Md62IsTargetPosAlready]
  [PosTolr] -> Subsystem16/5(Tolr)
  [Md61Calib] -> Subsystem/14(Md61Calib)
  [Md62Calib] -> Subsystem/15(Md62Calib)
  [Md61IsTargetPos] -> Subsystem1/43(Md61IsTargetPos)
  [Md62IsTargetPos] -> Subsystem1/44(Md62IsTargetPos)
  [Md61IsTargetPosAlready] -> Subsystem1/45(Md61IsTargetPosAlready)
  [Md61IsTargetPosZone] -> Subsystem1/47(Md61IsTargetPosZone)
  [Md62IsTargetPosAlready] -> Subsystem1/46(Md62IsTargetPosAlready)
  [Md62IsTargetPosZone] -> Subsystem1/48(Md62IsTargetPosZone)
  VIPLExitR2LBkReclnUpwdDnwdTrgtPosCalib_TrgtPosArray_read/1 -> [Md27Calib]
  Md27SecRwLtStBkReclnTrgtPosCalib_TrgtPosArray_read/1 -> [Md14Calib]
  [Md14Calib] -> Subsystem17/3(CalibArray)
  [Pos] -> Subsystem17/2(Pos)
  [PosV] -> Subsystem17/1(PosV)
  [PosTolr] -> Subsystem17/5(Tolr)
  [PosDelta] -> Subsystem17/4(Delta)
  Subsystem17/1(IsPos) -> [Md14IsTargetPos]
  Subsystem17/2(IsPosZone) -> [Md14IsTargetPosZone]
  Subsystem17/3(IsPosAlready) -> [Md14IsTargetPosAlready]
  [Md14IsTargetPos] -> Subsystem1/1(Md14IsTargetPos)
  [Md14IsTargetPosZone] -> Subsystem1/2(Md14IsTargetPosZone)
  [Md14IsTargetPosAlready] -> Subsystem1/3(Md14IsTargetPosAlready)

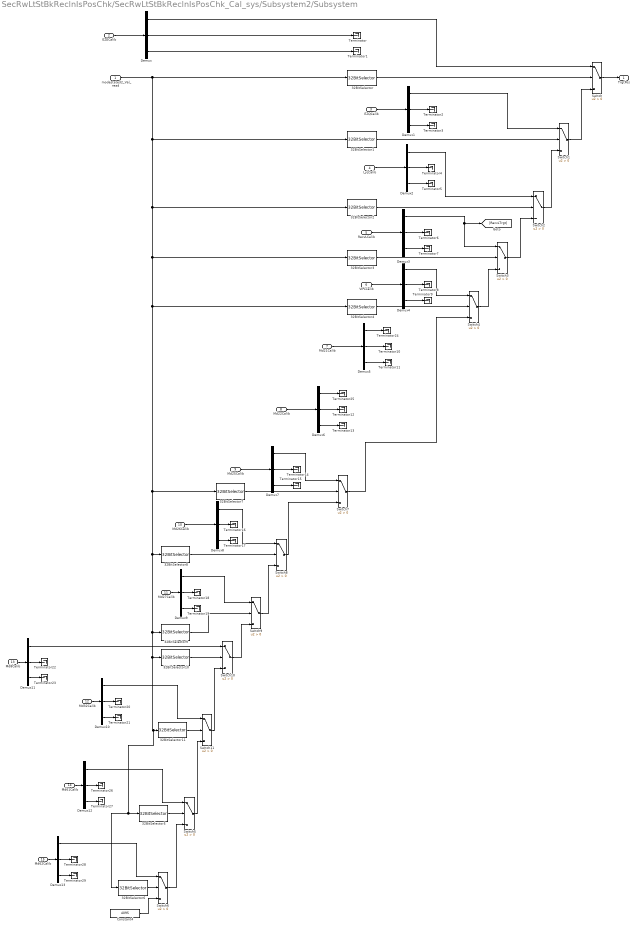
== system SecRwLtStBkReclnIsPosChk/SecRwLtStBkReclnIsPosChk_Cal_sys/Subsystem2/Subsystem ==
  modestate32_Val_read : Inport
  EZECalib : Inport  Port=2
  EZQCalib : Inport  Port=3
  LyLCalib : Inport  Port=4
  RecvLCalib : Inport  Port=5
  VIPLCalib : Inport  Port=6
  Md21Calib : Inport  Port=7
  Md22Calib : Inport  Port=8
  Md25Calib : Inport  Port=9
  Md26Calib : Inport  Port=10
  Md27Calib : Inport  Port=11
  Md32Calib : Inport  Port=12
  Md8Calib : Inport  Port=13
  Md61Calib : Inport  Port=14
  Md62Calib : Inport  Port=15
  32BitSelector : StIsPosChkLib/32BitSelector  BitNum=0
  32BitSelector1 : StIsPosChkLib/32BitSelector  BitNum=3
  32BitSelector10 : StIsPosChkLib/32BitSelector  BitNum=7
  32BitSelector11 : StIsPosChkLib/32BitSelector  BitNum=31
  32BitSelector2 : StIsPosChkLib/32BitSelector  BitNum=13
  32BitSelector3 : StIsPosChkLib/32BitSelector  BitNum=10
  32BitSelector4 : StIsPosChkLib/32BitSelector  BitNum=9
  32BitSelector5 : StIsPosChkLib/32BitSelector  BitNum=5
  32BitSelector6 : StIsPosChkLib/32BitSelector  BitNum=6
  32BitSelector7 : StIsPosChkLib/32BitSelector  BitNum=24
  32BitSelector8 : StIsPosChkLib/32BitSelector  BitNum=25
  32BitSelector9 : StIsPosChkLib/32BitSelector  BitNum=26
  Constant4 : Constant  Value=4095  OutDataTypeStr=uint16
  Demux{,1..13} (14 alike) : Demux  Outputs=3
  Switch{,1..11} (12 alike) : Switch  Criteria=u2 > Threshold  SaturateOnIntegerOverflow=off  InputSameDT=off
  Terminator{,1..29} (30 alike) : Terminator
  TrgtPos : Outport  VectorParamsAs1DForOutWhenUnconnected=off
      settings: EnsureOutportIsVirtual=on
  wires:
  32BitSelector/1 -> Switch/2
  Demux/1 -> Switch/1
  Demux/3 -> Terminator1/1
  Demux/2 -> Terminator/1
  EZECalib/1 -> Demux/1
  EZQCalib/1 -> Demux1/1
  Demux1/2 -> Terminator2/1
  Demux1/3 -> Terminator3/1
  Demux1/1 -> Switch1/1
  Switch/1 -> TrgtPos/1
  Switch1/1 -> Switch/3
  32BitSelector1/1 -> Switch1/2
  Switch2/1 -> Switch1/3
  Switch3/1 -> Switch2/3
  Switch4/1 -> Switch3/3
  32BitSelector2/1 -> Switch2/2
  32BitSelector3/1 -> Switch3/2
  32BitSelector4/1 -> Switch4/2
  Demux2/1 -> Switch2/1
  Demux2/3 -> Terminator5/1
  Demux2/2 -> Terminator4/1
  LyLCalib/1 -> Demux2/1
  RecvLCalib/1 -> Demux3/1
  Demux3/2 -> Terminator6/1
  Demux3/3 -> Terminator7/1
  Demux4/1 -> Switch4/1
  Demux4/3 -> Terminator9/1
  Demux4/2 -> Terminator8/1
  VIPLCalib/1 -> Demux4/1
  Md21Calib/1 -> Demux5/1
  Demux5/2 -> Terminator10/1
  Demux5/3 -> Terminator11/1
  Demux5/1 -> Terminator24/1
  modestate32_Val_read/1 -> 32BitSelector/1, 32BitSelector1/1, 32BitSelector2/1, 32BitSelector3/1, 32BitSelector5/1, 32BitSelector6/1, 32BitSelector11/1, 32BitSelector10/1, 32BitSelector9/1, 32BitSelector8/1, 32BitSelector7/1, 32BitSelector4/1
  Demux6/3 -> Terminator13/1
  Demux6/2 -> Terminator12/1
  Md22Calib/1 -> Demux6/1
  Md25Calib/1 -> Demux7/1
  Demux7/2 -> Terminator14/1
  Demux7/3 -> Terminator15/1
  Demux7/1 -> Switch7/1
  32BitSelector7/1 -> Switch7/2
  Demux8/1 -> Switch8/1
  Demux8/3 -> Terminator17/1
  Demux8/2 -> Terminator16/1
  Md26Calib/1 -> Demux8/1
  Switch7/1 -> Switch4/3
  Switch8/1 -> Switch7/3
  Md27Calib/1 -> Demux9/1
  Demux9/2 -> Terminator18/1
  Demux9/3 -> Terminator19/1
  Demux9/1 -> Switch9/1
  Switch9/1 -> Switch8/3
  32BitSelector8/1 -> Switch8/2
  32BitSelector9/1 -> Switch9/2
  Demux3/1 -> [RecvLTrgt], Switch3/1
  Switch10/1 -> Switch9/3
  Demux11/1 -> Switch10/1
  32BitSelector10/1 -> Switch10/2
  Switch11/1 -> Switch10/3
  32BitSelector11/1 -> Switch11/2
  Demux10/1 -> Switch11/1
  Demux10/3 -> Terminator21/1
  Demux10/2 -> Terminator20/1
  Md32Calib/1 -> Demux10/1
  Md8Calib/1 -> Demux11/1
  Demux11/2 -> Terminator22/1
  Demux11/3 -> Terminator23/1
  Demux6/1 -> Terminator25/1
  Switch5/1 -> Switch11/3
  Switch6/1 -> Switch5/3
  32BitSelector5/1 -> Switch5/2
  32BitSelector6/1 -> Switch6/2
  Constant4/1 -> Switch6/3
  Md61Calib/1 -> Demux12/1
  Demux12/2 -> Terminator26/1
  Demux12/3 -> Terminator27/1
  Demux12/1 -> Switch5/1
  Demux13/1 -> Switch6/1
  Demux13/3 -> Terminator29/1
  Demux13/2 -> Terminator28/1
  Md62Calib/1 -> Demux13/1
